simulink model "motor_unit"  (Simulink 7.8)
settings: Solver=ode14x  StartTime=0.0  StopTime=1  FixedStep=0.001  RelTol=1e-3
InitFcn:
  | [A tau T] = emg_filter()
  | [A_twitch T_twitch tau_twitch P e] = twitch_filter()
  |  [mag1 mag2 A_rise A_fall T] = get_active_function_coeff()
  | set_trfcn()
StopFcn:
  | incrementVars('motor_unit')
values from neighbouring files (symbols this model uses):
  A = exp(-T/tau)    [emg_filter.m]    (also in twitch_filter.m = [1 -2*A_twitch A_twitch^2] * P * e * A_twitch / tau_twitch)
  A_rise = exp(-T/t_rise)    [get_active_function_coeff.m]    (also in set_mu.m; set_mu_spasticity.m; set_trfcn.m)
  mag1 = 318144    [get_active_function_coeff.m]    (also in set_mu.m; set_mu_spasticity.m; set_trfcn.m)
  mag2 = 45845    [get_active_function_coeff.m]    (also in set_mu.m; set_mu_spasticity.m; set_trfcn.m)
  T = 1/1024    (= 0.0009765625)    [emg_filter.m]    (also in get_active_function_coeff.m = 0.001; set_mu.m = 0.001; set_mu_spasticity.m = 0.001; set_trfcn.m = 0.001)
  tau = 0.008    [emg_filter.m]
undefined symbols (not defined in the file or in its folder): dfilt, fdesignblkfcn, gcbh
libraries: cstblocks x25, simulink x11, dsparch4 x3
settings Model: Creator=minos_niu  LastModifiedBy=PXI_BBDL
settings DebuggingCC: FcnCallInpInsideContextMsg=Use local settings

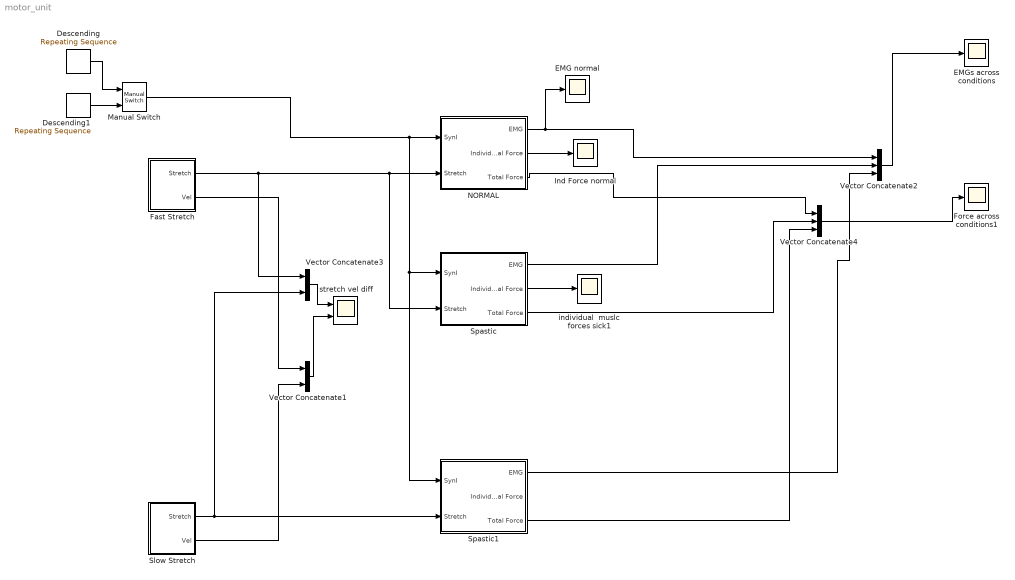
== system motor_unit ==
  Descending : simulink/Sources/Repeating Sequence  rep_seq_t=[0 0.5 1]  rep_seq_y=[0 200 200]*1
  Descending1 : simulink/Sources/Repeating Sequence  rep_seq_t=[0 0.5 1]  rep_seq_y=[0 200 200]*0
  EMG normal : Scope
      settings: TickLabels=on  TimeRange=1  YMin=-1000  YMax=5000  SaveName=ScopeData24
  EMGs across conditions : Scope
      settings: TickLabels=on  TimeRange=1  YMin=-1000  YMax=5000  SaveName=ScopeData6
  Fast Stretch : Subsystem
  Force across conditions1 : Scope
      settings: TickLabels=on  TimeRange=1  YMin=-1000  YMax=5000  SaveName=ScopeData5
  Ind Force normal : Scope
      settings: TickLabels=on  TimeRange=1  YMin=0  YMax=9e+09  SaveName=ScopeData21
  Manual Switch : simulink/Signal Routing/Manual Switch  sw=0  action=0  varsize=off
  NORMAL : Subsystem
  Slow Stretch : Subsystem
  Spastic : Subsystem
  Spastic1 : Subsystem
  Vector Concatenate1 : Concatenate  Mode=Vector
  Vector Concatenate2 : Concatenate  NumInputs=3  Mode=Vector
  Vector Concatenate3 : Concatenate  Mode=Vector
  Vector Concatenate4 : Concatenate  NumInputs=3  Mode=Vector
  individual  muslc forces sick1 : Scope
      settings: TickLabels=on  TimeRange=1  YMin=0  YMax=1.4e+10  SaveName=ScopeData8
  stretch vel diff : Scope  NumInputPorts=2
      settings: TickLabels=on  TimeRange=1  YMin=-5~-5  YMax=5~5  SaveName=ScopeData41
  wires:
  Spastic/1(EMG) -> Vector Concatenate2/2
  NORMAL/1(EMG) -> Vector Concatenate2/1, EMG normal/1
  NORMAL/3(Total Force) -> Vector Concatenate4/1
  Spastic/2(Individual Force) -> individual  muslc forces sick1/1
  Spastic/3(Total Force) -> Vector Concatenate4/2
  Vector Concatenate4/1 -> Force across conditions1/1
  Vector Concatenate2/1 -> EMGs across conditions/1
  Vector Concatenate1/1 -> stretch vel diff/2
  Vector Concatenate3/1 -> stretch vel diff/1
  Fast Stretch/1(Stretch) -> NORMAL/2(Stretch), Spastic/2(Stretch), Vector Concatenate3/1
  Slow Stretch/1(Stretch) -> Spastic1/2(Stretch), Vector Concatenate3/2
  Spastic1/1(EMG) -> Vector Concatenate2/3
  Fast Stretch/2(Vel) -> Vector Concatenate1/1
  Slow Stretch/2(Vel) -> Vector Concatenate1/2
  NORMAL/2(Individual Force) -> Ind Force normal/1
  Spastic1/3(Total Force) -> Vector Concatenate4/3
  Manual Switch/1 -> NORMAL/1(SynI), Spastic/1(SynI), Spastic1/1(SynI)
  Descending/1 -> Manual Switch/1
  Descending1/1 -> Manual Switch/2

== system motor_unit/Fast Stretch ==
  Discrete Derivative : simulink/Discrete/Discrete Derivative  gainval=1.0  ICPrevScaledInput=0.0  InputProcessing=Inherited  OutMin=[]  OutMax=[]  OutDataType=fixdt(1, 16)  OutScaling=2^-10  DoSatur=off
  Manual Switch : simulink/Signal Routing/Manual Switch  sw=0  action=0  varsize=off
  muscle stretch : simulink/Sources/Repeating Sequence  rep_seq_t=[0 0.25 0.8 1.5]  rep_seq_y=[1 1.00 1.0 1.0]
  muscle stretch1 : simulink/Sources/Repeating Sequence  rep_seq_t=[0 0.25 0.8 1.5]  rep_seq_y=[1 1.00 1.5 1.5]
  Stretch : Outport
  Vel : Outport  Port=2
  wires:
  Discrete Derivative/1 -> Vel/1
  Manual Switch/1 -> Discrete Derivative/1, Stretch/1
  muscle stretch/1 -> Manual Switch/1
  muscle stretch1/1 -> Manual Switch/2

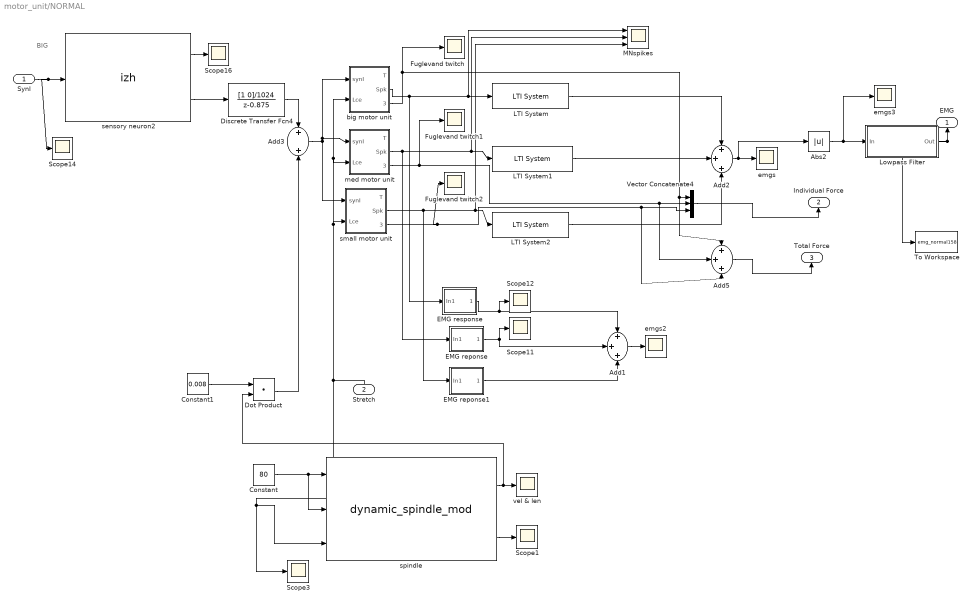
== system motor_unit/NORMAL ==
  note: BIG
  SynI : Inport
  Stretch : Inport  Port=2
  Abs2 : Abs
  Add1 : Sum  Inputs=+++
  Add2 : Sum  Inputs=+++
  Add3 : Sum
  Add5 : Sum  Inputs=+++
  Constant : Constant  Value=80
  Constant1 : Constant  Value=0.008
  Discrete Transfer Fcn4 : DiscreteTransferFcn  Numerator=[1 0]/1024  Denominator=[1 -0.875]  SampleTime=0.001
  Dot Product : DotProduct  InputSameDT=on  OutDataTypeStr=Inherit: Inherit via internal rule
  EMG reponse : Subsystem
  EMG reponse1 : Subsystem
  EMG response : Subsystem
  Fuglevand twitch : Scope
      settings: YMin=0  YMax=225
  Fuglevand twitch1 : Scope
      settings: YMin=0  YMax=225  SaveName=ScopeData27
  Fuglevand twitch2 : Scope
      settings: YMin=0  YMax=225  SaveName=ScopeData28
  LTI System : cstblocks/LTI System  sys=zpk([0], [A A], 2*T*A, T) - zpk([0 -A], [A A A], T^2*A/tau, T)  IC=[]
  LTI System1 : cstblocks/LTI System  sys=zpk([0], [A A], 2*T*A, T) - zpk([0 -A], [A A A], T^2*A/tau, T)  IC=[]
  LTI System2 : cstblocks/LTI System  sys=zpk([0], [A A], 2*T*A, T) - zpk([0 -A], [A A A], T^2*A/tau, T)  IC=[]
  Lowpass Filter : Subsystem  DialogController=fdesignblkfcn  DialogControllerArgs=DataTag1  InitFcn=fdesignblkfcn(gcbh, {'InitFcn'});
      settings: CopyFcn=fdesignblkfcn(gcbh, {'CopyFcn'});
      mask Type: Lowpass Filter
      mask Description: Design a lowpass filter
      mask Help: helpview(mapfilelocation('dsp'), 'dsplowpassfilter');
      mask Display: disp('Lowpass')
  MNspikes : Scope  NumInputPorts=3
      settings: YMin=0~-5~-5  YMax=225~5~5  SaveName=ScopeData2
  Scope{1,3,11..12,14,16} (6 alike) : Scope
      Scope1 settings: TimeRange=1  SaveName=ScopeData17
      Scope11 settings: SaveName=ScopeData9
      Scope12 settings: SaveName=ScopeData13
      Scope14 settings: YMin=0  YMax=225  SaveName=ScopeData14
      Scope16 settings: SaveName=ScopeData16
      Scope3 settings: SaveName=ScopeData18
  To Workspace : ToWorkspace  VariableName=emg_normal158  SampleTime=-1  SaveFormat=Structure With Time
  Vector Concatenate4 : Concatenate  NumInputs=3  Mode=Vector
  big motor unit : Subsystem
  emgs : Scope
      settings: YMin=0  YMax=225
  emgs2 : Scope
      settings: TimeRange=1  YMin=-0.03  YMax=0.03  SaveName=ScopeData15
  emgs3 : Scope
      settings: YMin=0  YMax=225  SaveName=ScopeData3
  med motor unit : Subsystem
  sensory neuron2 : S-Function  FunctionName=izh  Parameters=[0.02 0.2 -65.0 6.0 30.0 3.0] [-70.0 -14.0]  EnableBusSupport=off
      mask Display:
      | port_label('input', 1, 'syn curr');
      | port_label('output', 1, 'action potential');
      | port_label('output', 2, 'spike');
      | disp('Izhi Neuron \n(S-Function)')
  small motor unit : Subsystem
  spindle : S-Function  FunctionName=dynamic_spindle_mod  Parameters=[10.4649 10.4649 10.4649] [0.1127 0.1623 0.1623] [0.0605 0.0822 0.0822] [0.2356 -0.046 -0.069] [0 0 0] [0.0289 0.0636 0.0954] [1 0.7 0.7] [1 0.92 0.92] [20000 10000 10000] [20000 7250 7250] [0.3 0.3 0.3] [0.46 0.46 0.46] [0.04 0.04 0.04] [0.76 0.76 0.76] [1 0.04 0.04] [0.192 0.185 0.0001] [0.0002 0.0002 0.0002] [1 0.5 1] [1]  EnableBusSupport=off
      mask Display:
      | port_label('input', 1, 'gamma dynamic');
      | port_label('input', 2, 'gamma static');
      | port_label('input', 3, 'Lce(L0)');
      | port_label('output',1,'Ia');
      | port_label('output',2,'II');
      | disp('Muscle Spindle \n(S-Function)')
  vel & len : Scope
      settings: SaveName=ScopeData12
  EMG : Outport
  Individual Force : Outport  Port=2
  Total Force : Outport  Port=3
  wires:
  Abs2/1 -> Lowpass Filter/1(In), emgs3/1
  Lowpass Filter/1(Out) -> To Workspace/1, EMG/1
  Add3/1 -> big motor unit/1(synI), med motor unit/1(synI), small motor unit/1(synI)
  Discrete Transfer Fcn4/1 -> Add3/1
  Dot Product/1 -> Add3/2
  Constant1/1 -> Dot Product/1
  Stretch/1 -> Scope3/1, spindle/3, big motor unit/2(Lce), med motor unit/2(Lce), small motor unit/2(Lce)
  spindle/2 -> Scope1/1
  spindle/1 -> vel & len/1, Dot Product/2
  Constant/1 -> spindle/1, spindle/2
  EMG reponse1/1(Out1) -> Add1/3
  Add1/1 -> emgs2/1
  big motor unit/2(Spk) -> EMG response/1(In1), LTI System/1, MNspikes/1
  LTI System2/1 -> Add2/3
  LTI System1/1 -> Add2/2
  LTI System/1 -> Add2/1
  Add2/1 -> emgs/1, Abs2/1
  sensory neuron2/2 -> Discrete Transfer Fcn4/1
  Add5/1 -> Total Force/1
  sensory neuron2/1 -> Scope16/1
  SynI/1 -> Scope14/1, sensory neuron2/1
  EMG response/1(Out1) -> Scope12/1, Add1/1
  EMG reponse/1(Out1) -> Scope11/1, Add1/2
  Vector Concatenate4/1 -> Individual Force/1
  big motor unit/3(Fubglevant  twitch normal) -> Fuglevand twitch/1, Vector Concatenate4/1, Add5/1
  med motor unit/2(Spk) -> EMG reponse/1(In1), LTI System1/1, MNspikes/2
  small motor unit/2(Spk) -> EMG reponse1/1(In1), LTI System2/1, MNspikes/3
  med motor unit/3(Fubglevant  twitch normal) -> Fuglevand twitch1/1, Vector Concatenate4/2, Add5/2
  small motor unit/3(Fubglevant  twitch normal) -> Fuglevand twitch2/1, Vector Concatenate4/3, Add5/3

== system motor_unit/Slow Stretch ==
  Discrete Derivative : simulink/Discrete/Discrete Derivative  gainval=1.0  ICPrevScaledInput=0.0  InputProcessing=Inherited  OutMin=[]  OutMax=[]  OutDataType=fixdt(1, 16)  OutScaling=2^-10  DoSatur=off
  Manual Switch : simulink/Signal Routing/Manual Switch  sw=0  action=0  varsize=off
  muscle stretch : simulink/Sources/Repeating Sequence  rep_seq_t=[0 0.25 0.8 1.5]  rep_seq_y=[1 1.00 1.0 1.0]
  muscle stretch1 : simulink/Sources/Repeating Sequence  rep_seq_t=[0 0.25 0.65 1.5]  rep_seq_y=[1 1.00 1.5 1.5]
  Stretch : Outport
  Vel : Outport  Port=2
  wires:
  muscle stretch1/1 -> Manual Switch/2
  muscle stretch/1 -> Manual Switch/1
  Manual Switch/1 -> Stretch/1, Discrete Derivative/1
  Discrete Derivative/1 -> Vel/1

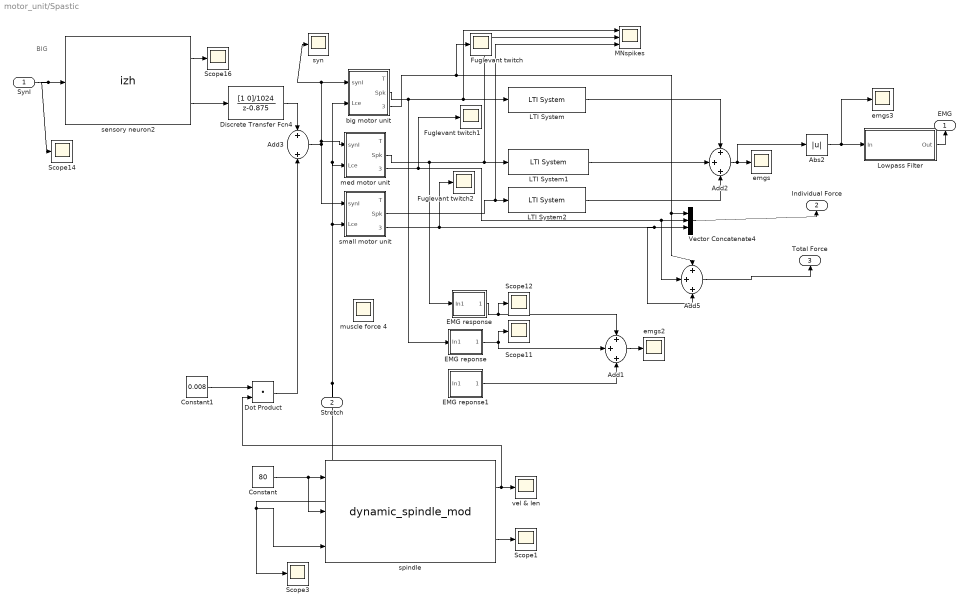
== system motor_unit/Spastic ==
  note: BIG
  SynI : Inport
  Stretch : Inport  Port=2
  " Fuglevant twitch" : Scope
      settings: YMin=0  YMax=225  SaveName=ScopeData26
  " Fuglevant twitch1" : Scope
      settings: YMin=0  YMax=225  SaveName=ScopeData4
  " Fuglevant twitch2" : Scope
      settings: YMin=0  YMax=225  SaveName=ScopeData11
  Abs2 : Abs
  Add1 : Sum  Inputs=+++
  Add2 : Sum  Inputs=+++
  Add3 : Sum
  Add5 : Sum  Inputs=+++
  Constant : Constant  Value=80
  Constant1 : Constant  Value=0.008
  Discrete Transfer Fcn4 : DiscreteTransferFcn  Numerator=[1 0]/1024  Denominator=[1 -0.875]  SampleTime=0.001
  Dot Product : DotProduct  InputSameDT=on  OutDataTypeStr=Inherit: Inherit via internal rule
  EMG reponse : Subsystem
  EMG reponse1 : Subsystem
  EMG response : Subsystem
  LTI System : cstblocks/LTI System  sys=zpk([0], [A A], 2*T*A, T) - zpk([0 -A], [A A A], T^2*A/tau, T)  IC=[]
  LTI System1 : cstblocks/LTI System  sys=zpk([0], [A A], 2*T*A, T) - zpk([0 -A], [A A A], T^2*A/tau, T)  IC=[]
  LTI System2 : cstblocks/LTI System  sys=zpk([0], [A A], 2*T*A, T) - zpk([0 -A], [A A A], T^2*A/tau, T)  IC=[]
  Lowpass Filter : Subsystem  DialogController=fdesignblkfcn  DialogControllerArgs=DataTag4  InitFcn=fdesignblkfcn(gcbh, {'InitFcn'});
      settings: CopyFcn=fdesignblkfcn(gcbh, {'CopyFcn'});
      mask Type: Lowpass Filter
      mask Description: Design a lowpass filter
      mask Help: helpview(mapfilelocation('dsp'), 'dsplowpassfilter');
      mask Display: disp('Lowpass')
  MNspikes : Scope  NumInputPorts=3
      settings: YMin=0~-5~-5  YMax=225~5~5  SaveName=ScopeData20
  Scope{1,3,11..12,14,16} (6 alike) : Scope
      Scope1 settings: TimeRange=1  SaveName=ScopeData17
      Scope11 settings: SaveName=ScopeData9
      Scope12 settings: SaveName=ScopeData13
      Scope14 settings: YMin=0  YMax=225  SaveName=ScopeData14
      Scope16 settings: SaveName=ScopeData16
      Scope3 settings: SaveName=ScopeData18
  Vector Concatenate4 : Concatenate  NumInputs=3  Mode=Vector
  big motor unit : Subsystem
  emgs : Scope
      settings: YMin=0  YMax=225
  emgs2 : Scope
      settings: TimeRange=1  YMin=-0.03  YMax=0.03  SaveName=ScopeData15
  emgs3 : Scope
      settings: YMin=0  YMax=225  SaveName=ScopeData3
  med motor unit : Subsystem
  muscle force 4 : Scope
      settings: YMin=0  YMax=225  SaveName=ScopeData7
  sensory neuron2 : S-Function  FunctionName=izh  Parameters=[0.02 0.2 -65.0 6.0 30.0 3.0] [-70.0 -14.0]  EnableBusSupport=off
      mask Display:
      | port_label('input', 1, 'syn curr');
      | port_label('output', 1, 'action potential');
      | port_label('output', 2, 'spike');
      | disp('Izhi Neuron \n(S-Function)')
  small motor unit : Subsystem
  spindle : S-Function  FunctionName=dynamic_spindle_mod  Parameters=[10.4649 10.4649 10.4649] [0.1127 0.1623 0.1623] [0.0605 0.0822 0.0822] [0.2356 -0.046 -0.069] [0 0 0] [0.0289 0.0636 0.0954] [1 0.7 0.7] [1 0.92 0.92] [20000 10000 10000] [20000 7250 7250] [0.3 0.3 0.3] [0.46 0.46 0.46] [0.04 0.04 0.04] [0.76 0.76 0.76] [1 0.04 0.04] [0.192 0.185 0.0001] [0.0002 0.0002 0.0002] [1 0.5 1] [1]  EnableBusSupport=off
      mask Display:
      | port_label('input', 1, 'gamma dynamic');
      | port_label('input', 2, 'gamma static');
      | port_label('input', 3, 'Lce(L0)');
      | port_label('output',1,'Ia');
      | port_label('output',2,'II');
      | disp('Muscle Spindle \n(S-Function)')
  syn : Scope
      settings: YMin=0  YMax=225  SaveName=ScopeData25
  vel & len : Scope
      settings: SaveName=ScopeData12
  EMG : Outport
  Individual Force : Outport  Port=2
  Total Force : Outport  Port=3
  wires:
  Vector Concatenate4/1 -> Individual Force/1
  EMG reponse/1(Out1) -> Add1/2, Scope11/1
  EMG response/1(Out1) -> Add1/1, Scope12/1
  SynI/1 -> sensory neuron2/1, Scope14/1
  sensory neuron2/1 -> Scope16/1
  Add5/1 -> Total Force/1
  sensory neuron2/2 -> Discrete Transfer Fcn4/1
  Add2/1 -> Abs2/1, emgs/1
  LTI System/1 -> Add2/1
  LTI System1/1 -> Add2/2
  LTI System2/1 -> Add2/3
  big motor unit/2(Spk) -> EMG reponse/1(In1), LTI System/1, MNspikes/1
  med motor unit/2(Spk) -> EMG response/1(In1), LTI System1/1, MNspikes/2
  Add1/1 -> emgs2/1
  EMG reponse1/1(Out1) -> Add1/3
  Constant/1 -> spindle/2, spindle/1
  spindle/1 -> Dot Product/2, vel & len/1
  spindle/2 -> Scope1/1
  Stretch/1 -> spindle/3, Scope3/1, big motor unit/2(Lce), med motor unit/2(Lce), small motor unit/2(Lce)
  Constant1/1 -> Dot Product/1
  Dot Product/1 -> Add3/2
  Discrete Transfer Fcn4/1 -> Add3/1
  Add3/1 -> big motor unit/1(synI), syn/1, med motor unit/1(synI), small motor unit/1(synI)
  Lowpass Filter/1(Out) -> EMG/1
  Abs2/1 -> emgs3/1, Lowpass Filter/1(In)
  med motor unit/3(Fubglevant  twitch) -> Vector Concatenate4/2, Add5/2, " Fuglevant twitch1"/1
  big motor unit/3(Fubglevant  twitch) -> " Fuglevant twitch"/1, Vector Concatenate4/1, Add5/1
  small motor unit/3(Fubglevant  twitch) -> Vector Concatenate4/3, Add5/3, " Fuglevant twitch2"/1
  small motor unit/2(Spk) -> LTI System2/1, MNspikes/3

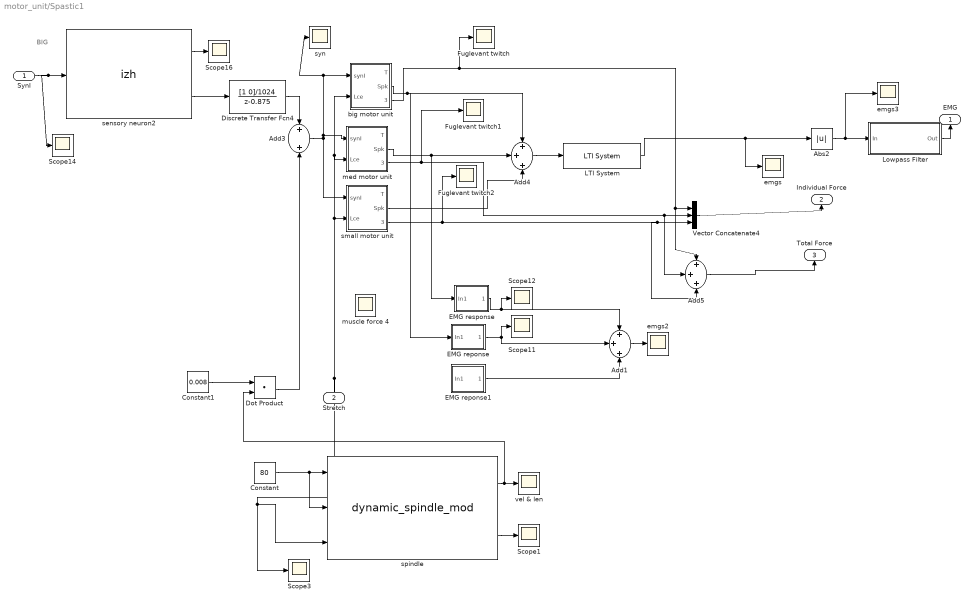
== system motor_unit/Spastic1 ==
  note: BIG
  SynI : Inport
  Stretch : Inport  Port=2
  " Fuglevant twitch" : Scope
      settings: YMin=0  YMax=225  SaveName=ScopeData26
  " Fuglevant twitch1" : Scope
      settings: YMin=0  YMax=225  SaveName=ScopeData4
  " Fuglevant twitch2" : Scope
      settings: YMin=0  YMax=225  SaveName=ScopeData11
  Abs2 : Abs
  Add1 : Sum  Inputs=+++
  Add3 : Sum
  Add4 : Sum  Inputs=+++
  Add5 : Sum  Inputs=+++
  Constant : Constant  Value=80
  Constant1 : Constant  Value=0.008
  Discrete Transfer Fcn4 : DiscreteTransferFcn  Numerator=[1 0]/1024  Denominator=[1 -0.875]  SampleTime=0.001
  Dot Product : DotProduct  InputSameDT=on  OutDataTypeStr=Inherit: Inherit via internal rule
  EMG reponse : Subsystem
  EMG reponse1 : Subsystem
  EMG response : Subsystem
  LTI System : cstblocks/LTI System  sys=zpk([0], [A A], 2*T*A, T) - zpk([0 -A], [A A A], T^2*A/tau, T)  IC=[]
  Lowpass Filter : Subsystem  DialogController=fdesignblkfcn  DialogControllerArgs=DataTag7  InitFcn=fdesignblkfcn(gcbh, {'InitFcn'});
      settings: CopyFcn=fdesignblkfcn(gcbh, {'CopyFcn'});
      mask Type: Lowpass Filter
      mask Description: Design a lowpass filter
      mask Help: helpview(mapfilelocation('dsp'), 'dsplowpassfilter');
      mask Display: disp('Lowpass')
  Scope{1,3,11..12,14,16} (6 alike) : Scope
      Scope1 settings: TimeRange=1  SaveName=ScopeData17
      Scope11 settings: SaveName=ScopeData9
      Scope12 settings: SaveName=ScopeData13
      Scope14 settings: YMin=0  YMax=225  SaveName=ScopeData14
      Scope16 settings: SaveName=ScopeData16
      Scope3 settings: SaveName=ScopeData18
  Vector Concatenate4 : Concatenate  NumInputs=3  Mode=Vector
  big motor unit : Subsystem
  emgs : Scope
      settings: YMin=0  YMax=225
  emgs2 : Scope
      settings: TimeRange=1  YMin=-0.03  YMax=0.03  SaveName=ScopeData15
  emgs3 : Scope
      settings: YMin=0  YMax=225  SaveName=ScopeData3
  med motor unit : Subsystem
  muscle force 4 : Scope
      settings: YMin=0  YMax=225  SaveName=ScopeData7
  sensory neuron2 : S-Function  FunctionName=izh  Parameters=[0.02 0.2 -65.0 6.0 30.0 3.0] [-70.0 -14.0]  EnableBusSupport=off
      mask Display:
      | port_label('input', 1, 'syn curr');
      | port_label('output', 1, 'action potential');
      | port_label('output', 2, 'spike');
      | disp('Izhi Neuron \n(S-Function)')
  small motor unit : Subsystem
  spindle : S-Function  FunctionName=dynamic_spindle_mod  Parameters=[10.4649 10.4649 10.4649] [0.1127 0.1623 0.1623] [0.0605 0.0822 0.0822] [0.2356 -0.046 -0.069] [0 0 0] [0.0289 0.0636 0.0954] [1 0.7 0.7] [1 0.92 0.92] [20000 10000 10000] [20000 7250 7250] [0.3 0.3 0.3] [0.46 0.46 0.46] [0.04 0.04 0.04] [0.76 0.76 0.76] [1 0.04 0.04] [0.192 0.185 0.0001] [0.0002 0.0002 0.0002] [1 0.5 1] [1]  EnableBusSupport=off
      mask Display:
      | port_label('input', 1, 'gamma dynamic');
      | port_label('input', 2, 'gamma static');
      | port_label('input', 3, 'Lce(L0)');
      | port_label('output',1,'Ia');
      | port_label('output',2,'II');
      | disp('Muscle Spindle \n(S-Function)')
  syn : Scope
      settings: YMin=0  YMax=225  SaveName=ScopeData25
  vel & len : Scope
      settings: SaveName=ScopeData12
  EMG : Outport
  Individual Force : Outport  Port=2
  Total Force : Outport  Port=3
  wires:
  small motor unit/2(Spk) -> Add4/3
  small motor unit/3(Fubglevant  twitch) -> " Fuglevant twitch2"/1, Add5/3, Vector Concatenate4/3
  big motor unit/3(Fubglevant  twitch) -> Add5/1, Vector Concatenate4/1, " Fuglevant twitch"/1
  med motor unit/3(Fubglevant  twitch) -> " Fuglevant twitch1"/1, Add5/2, Vector Concatenate4/2
  Abs2/1 -> Lowpass Filter/1(In), emgs3/1
  Lowpass Filter/1(Out) -> EMG/1
  Add3/1 -> small motor unit/1(synI), med motor unit/1(synI), syn/1, big motor unit/1(synI)
  Discrete Transfer Fcn4/1 -> Add3/1
  Dot Product/1 -> Add3/2
  Constant1/1 -> Dot Product/1
  Stretch/1 -> small motor unit/2(Lce), med motor unit/2(Lce), big motor unit/2(Lce), Scope3/1, spindle/3
  spindle/2 -> Scope1/1
  spindle/1 -> vel & len/1, Dot Product/2
  Constant/1 -> spindle/1, spindle/2
  EMG reponse1/1(Out1) -> Add1/3
  Add1/1 -> emgs2/1
  med motor unit/2(Spk) -> EMG response/1(In1), Add4/2
  big motor unit/2(Spk) -> EMG reponse/1(In1), Add4/1
  LTI System/1 -> emgs/1, Abs2/1
  sensory neuron2/2 -> Discrete Transfer Fcn4/1
  Add5/1 -> Total Force/1
  sensory neuron2/1 -> Scope16/1
  SynI/1 -> Scope14/1, sensory neuron2/1
  EMG response/1(Out1) -> Scope12/1, Add1/1
  EMG reponse/1(Out1) -> Scope11/1, Add1/2
  Vector Concatenate4/1 -> Individual Force/1
  Add4/1 -> LTI System/1

== system motor_unit/NORMAL/EMG reponse ==
  In1 : Inport
  Add1 : Sum
  Zero-Pole : ZeroPole  Zeros=[]  Poles=[-33 -33]  Gain=[2]
  Zero-Pole1 : ZeroPole  Zeros=[]  Poles=[-33 -33 -33]  Gain=[-2 * 33]
  Out1 : Outport
  wires:
  Zero-Pole/1 -> Add1/1
  Zero-Pole1/1 -> Add1/2
  Add1/1 -> Out1/1
  In1/1 -> Zero-Pole/1, Zero-Pole1/1

== system motor_unit/NORMAL/EMG reponse1 ==
  In1 : Inport
  Add1 : Sum
  Zero-Pole : ZeroPole  Zeros=[]  Poles=[-33 -33]  Gain=[2]
  Zero-Pole1 : ZeroPole  Zeros=[]  Poles=[-33 -33 -33]  Gain=[-2 * 33]
  Out1 : Outport
  wires:
  Zero-Pole/1 -> Add1/1
  Zero-Pole1/1 -> Add1/2
  Add1/1 -> Out1/1
  In1/1 -> Zero-Pole/1, Zero-Pole1/1

== system motor_unit/NORMAL/EMG response ==
  In1 : Inport
  Add2 : Sum
  Zero-Pole2 : ZeroPole  Zeros=[]  Poles=[-33 -33]  Gain=[2]
  Zero-Pole3 : ZeroPole  Zeros=[]  Poles=[-33 -33 -33]  Gain=[-2 * 33]
  Out1 : Outport
  wires:
  Zero-Pole3/1 -> Add2/2
  Zero-Pole2/1 -> Add2/1
  In1/1 -> Zero-Pole2/1, Zero-Pole3/1
  Add2/1 -> Out1/1

== system motor_unit/NORMAL/Lowpass Filter ==
  In : Inport
  Generated Filter Block : dsparch4/Digital Filter  Tag=BlockMethodSubSystem  TypePopup=FIR (all zeros)  IIRFiltStruct=Direct form II transposed  AllPoleFiltStruct=Direct form  FIRFiltStruct=Direct form  CoeffSource=Specify via dialog  NumCoeffs=[0.000821343113298559 0.000860441837741389 0.00116507777294478 0.00139896051971534 0.00148073798259756 0.00133051719232521 0.000881379928818246 9.39666659446496e-05 -0.00102427649336678 -0.00241508381296073 -0.00396005761838719 -0.00548791113381279 -0.00678957165103652 -0.0076430176358472 -0.00784363593055865 -0.00724034355165257 -0.005767373855361 -0.00347179427273649 -0.000526738025008324 0.00277189505493066 0.00602772399348037 0.00878384411363102 0.0105793849551558 0.0110144101671425 0.00981730876000813 0.00690368741433792 0.00241805574190362 -0.00324979313849789 -0.00947842883556182 -0.0154612118882062 -0.0202815328070714 -0.0230109852998383 -0.0228194406688834 -0.0190843479651619 -0.0114852033107793 -7.04588646032898e-05 0.0147140504913441 0.032040450344853 0.0507590050669597 0.0694980891161205 0.0867940010093986 0.101236365407667 0.111612741087645 0.117035389882844 0.117035389882844 0.111612741087645 0.101236365407667 0.0867940010093986 0.0694980891161205 0.0507590050669597 0.032040450344853 0.0147140504913441 -7.04588646032898e-05 -0.0114852033107793 -0.0190843479651619 -0.0228194406688834 -0.0230109852998383 -0.0202815328070714 -0.0154612118882062 -0.00947842883556182 -0.00324979313849789 0.00241805574190362 0.00690368741433792 0.00981730876000813 0.0110144101671425 0.0105793849551558 0.00878384411363102 0.00602772399348037 0.00277189505493066 -0.000526738025008324 -0.00347179427273649 -0.005767373855361 -0.00724034355165257 -0.00784363593055865 -0.0076430176358472 -0.00678957165103652 -0.00548791113381279 -0.00396005761838719 -0.00241508381296073 -0.00102427649336678 9.39666659446496e-05 0.000881379928818246 0.00133051719232521 0.00148073798259756 0.00139896051971534 0.00116507777294478 0.000860441837741389 0.000821343113298559]  DenCoeffs=[1 0.1]  BiQuadCoeffs=[1 0.3 0.4 1 0.1 0.2]  LatticeCoeffs=[0.2 0.4]  denIgnore=on  FiltPerSampPopup=One filter per frame  IC=0  ICnum=0  ICden=0  roundingMode=Floor  overflowMode=off  ScaleValues=1  scaleValueFracLength=14  stageInFracLength=15  stageOutFracLength=15  FilterSource=Specify via dialog  dfiltObjectName=dfilt.dffir([1 2 1])  InputProcessing=Columns as channels (frame based)
  Out : Outport
  wires:
  In/1 -> Generated Filter Block/1
  Generated Filter Block/1 -> Out/1

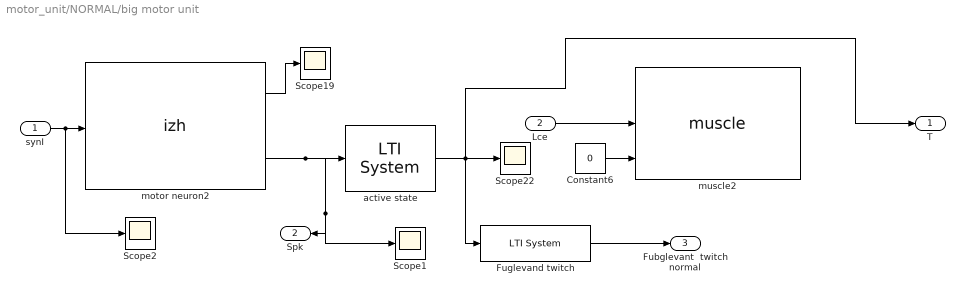
== system motor_unit/NORMAL/big motor unit ==
  synI : Inport
  Lce : Inport  Port=2
  Constant6 : Constant  Value=0
  Fuglevand twitch : cstblocks/LTI System  sys=zpk([0], [0.93941 0.93941], 1*2.7183*0.001*0.93941/0.016, 0.001)  IC=[]
  Scope{1..2,19,22} (4 alike) : Scope
      Scope1 settings: TimeRange=0.4  YMin=-1000  YMax=5000  SaveName=ScopeData10
      Scope19 settings: SaveName=ScopeData19
      Scope2 settings: SaveName=ScopeData29
      Scope22 settings: TimeRange=0.4  YMin=-1000  YMax=5000  SaveName=ScopeData22
  active state : cstblocks/LTI System  sys="0*zpk([0], 0.97531, 318144, T) + zpk([0], exp(-T/0.04),  mag2*8, T)"  IC=[]
  motor neuron2 : S-Function  FunctionName=izh  Parameters=[0.02 0.2 -65.0 6.0 30.0 0.45] [-70.0 -14.0]  EnableBusSupport=off
      mask Display:
      | port_label('input', 1, 'syn curr');
      | port_label('output', 1, 'action potential');
      | port_label('output', 2, 'spike');
      | disp('Izhi Neuron \n(S-Function)')
  muscle2 : S-Function  FunctionName=muscle  Parameters=[136.0 75.0 50.0] [0]  EnableBusSupport=off
      mask Display:
      | port_label('input', 1, 'Active state');
      | port_label('input', 2, 'length');
      | port_label('input', 3, 'vel');
      | port_label('output', 1, 'tension');
      | disp('muscle model \n(S-Function)');
  T : Outport
  Spk : Outport  Port=2
  Fubglevant  twitch normal : Outport  Port=3
  wires:
  Constant6/1 -> muscle2/3
  motor neuron2/1 -> Scope19/1
  active state/1 -> Scope22/1, T/1, Fuglevand twitch/1
  motor neuron2/2 -> active state/1, Spk/1, Scope1/1
  synI/1 -> motor neuron2/1, Scope2/1
  Lce/1 -> muscle2/2
  Fuglevand twitch/1 -> Fubglevant  twitch normal/1

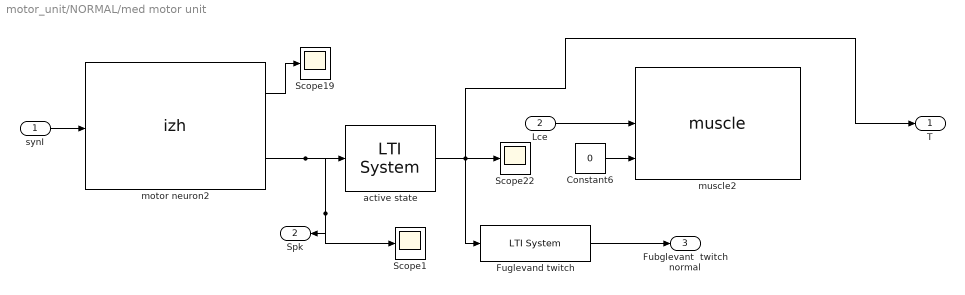
== system motor_unit/NORMAL/med motor unit ==
  synI : Inport
  Lce : Inport  Port=2
  Constant6 : Constant  Value=0
  Fuglevand twitch : cstblocks/LTI System  sys=zpk([0], [0.93941 0.93941], 1*2.7183*0.001*0.93941/0.016, 0.001)  IC=[]
  Scope1 : Scope
      settings: TimeRange=0.4  YMin=-1000  YMax=5000  SaveName=ScopeData10
  Scope19 : Scope
      settings: SaveName=ScopeData19
  Scope22 : Scope
      settings: TimeRange=0.4  YMin=-1000  YMax=5000  SaveName=ScopeData22
  active state : cstblocks/LTI System  sys="0*zpk([0], A_rise, mag1, T) + zpk([0], exp(-T/0.06),  mag2*3.5, T)"  IC=[]
  motor neuron2 : S-Function  FunctionName=izh  Parameters=[0.02 0.2 -65.0 6.0 30.0 0.50] [-70.0 -14.0]  EnableBusSupport=off
      mask Display:
      | port_label('input', 1, 'syn curr');
      | port_label('output', 1, 'action potential');
      | port_label('output', 2, 'spike');
      | disp('Izhi Neuron \n(S-Function)')
  muscle2 : S-Function  FunctionName=muscle  Parameters=[136.0 75.0 50.0] [0]  EnableBusSupport=off
      mask Display:
      | port_label('input', 1, 'Active state');
      | port_label('input', 2, 'length');
      | port_label('input', 3, 'vel');
      | port_label('output', 1, 'tension');
      | disp('muscle model \n(S-Function)');
  T : Outport
  Spk : Outport  Port=2
  Fubglevant  twitch normal : Outport  Port=3
  wires:
  Fuglevand twitch/1 -> Fubglevant  twitch normal/1
  Lce/1 -> muscle2/2
  synI/1 -> motor neuron2/1
  motor neuron2/2 -> Scope1/1, Spk/1, active state/1
  active state/1 -> Fuglevand twitch/1, T/1, Scope22/1
  motor neuron2/1 -> Scope19/1
  Constant6/1 -> muscle2/3

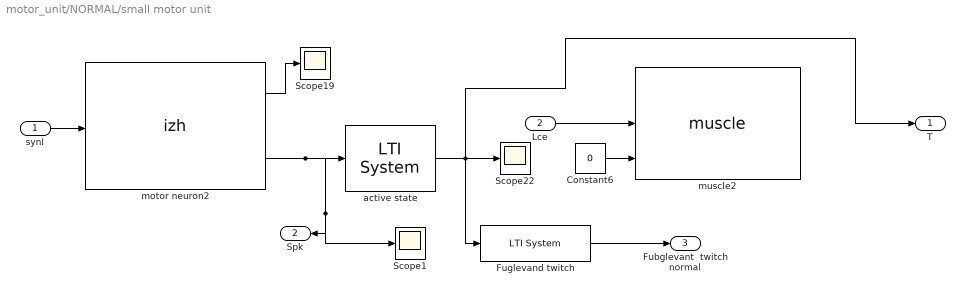
== system motor_unit/NORMAL/small motor unit ==
  synI : Inport
  Lce : Inport  Port=2
  Constant6 : Constant  Value=0
  Fuglevand twitch : cstblocks/LTI System  sys=zpk([0], [0.93941 0.93941], 1*2.7183*0.001*0.93941/0.016, 0.001)  IC=[]
  Scope1 : Scope
      settings: TimeRange=0.4  YMin=-1000  YMax=5000  SaveName=ScopeData10
  Scope19 : Scope
      settings: SaveName=ScopeData19
  Scope22 : Scope
      settings: TimeRange=0.4  YMin=-1000  YMax=5000  SaveName=ScopeData22
  active state : cstblocks/LTI System  sys=0*zpk([0], A_rise, mag1, T) + zpk([0], exp(-T/0.09), mag2*1, T)  IC=[]
  motor neuron2 : S-Function  FunctionName=izh  Parameters=[0.02 0.2 -65.0 6.0 30.0 0.55] [-70.0 -14.0]  EnableBusSupport=off
      mask Display:
      | port_label('input', 1, 'syn curr');
      | port_label('output', 1, 'action potential');
      | port_label('output', 2, 'spike');
      | disp('Izhi Neuron \n(S-Function)')
  muscle2 : S-Function  FunctionName=muscle  Parameters=[136.0 75.0 50.0] [0]  EnableBusSupport=off
      mask Display:
      | port_label('input', 1, 'Active state');
      | port_label('input', 2, 'length');
      | port_label('input', 3, 'vel');
      | port_label('output', 1, 'tension');
      | disp('muscle model \n(S-Function)');
  T : Outport
  Spk : Outport  Port=2
  Fubglevant  twitch normal : Outport  Port=3
  wires:
  Constant6/1 -> muscle2/3
  motor neuron2/1 -> Scope19/1
  active state/1 -> Scope22/1, T/1, Fuglevand twitch/1
  motor neuron2/2 -> active state/1, Spk/1, Scope1/1
  synI/1 -> motor neuron2/1
  Lce/1 -> muscle2/2
  Fuglevand twitch/1 -> Fubglevant  twitch normal/1

== system motor_unit/Spastic/EMG reponse ==
  In1 : Inport
  Add1 : Sum
  Zero-Pole : ZeroPole  Zeros=[]  Poles=[-33 -33]  Gain=[2]
  Zero-Pole1 : ZeroPole  Zeros=[]  Poles=[-33 -33 -33]  Gain=[-2 * 33]
  Out1 : Outport
  wires:
  In1/1 -> Zero-Pole1/1, Zero-Pole/1
  Add1/1 -> Out1/1
  Zero-Pole1/1 -> Add1/2
  Zero-Pole/1 -> Add1/1

== system motor_unit/Spastic/EMG reponse1 ==
  In1 : Inport
  Add1 : Sum
  Zero-Pole : ZeroPole  Zeros=[]  Poles=[-33 -33]  Gain=[2]
  Zero-Pole1 : ZeroPole  Zeros=[]  Poles=[-33 -33 -33]  Gain=[-2 * 33]
  Out1 : Outport
  wires:
  In1/1 -> Zero-Pole1/1, Zero-Pole/1
  Add1/1 -> Out1/1
  Zero-Pole1/1 -> Add1/2
  Zero-Pole/1 -> Add1/1

== system motor_unit/Spastic/EMG response ==
  In1 : Inport
  Add2 : Sum
  Zero-Pole2 : ZeroPole  Zeros=[]  Poles=[-33 -33]  Gain=[2]
  Zero-Pole3 : ZeroPole  Zeros=[]  Poles=[-33 -33 -33]  Gain=[-2 * 33]
  Out1 : Outport
  wires:
  Add2/1 -> Out1/1
  In1/1 -> Zero-Pole3/1, Zero-Pole2/1
  Zero-Pole2/1 -> Add2/1
  Zero-Pole3/1 -> Add2/2

== system motor_unit/Spastic/Lowpass Filter ==
  In : Inport
  Generated Filter Block : dsparch4/Digital Filter  Tag=BlockMethodSubSystem  TypePopup=FIR (all zeros)  IIRFiltStruct=Direct form II transposed  AllPoleFiltStruct=Direct form  FIRFiltStruct=Direct form  CoeffSource=Specify via dialog  NumCoeffs=[0.000821343113298559 0.000860441837741389 0.00116507777294478 0.00139896051971534 0.00148073798259756 0.00133051719232521 0.000881379928818246 9.39666659446496e-05 -0.00102427649336678 -0.00241508381296073 -0.00396005761838719 -0.00548791113381279 -0.00678957165103652 -0.0076430176358472 -0.00784363593055865 -0.00724034355165257 -0.005767373855361 -0.00347179427273649 -0.000526738025008324 0.00277189505493066 0.00602772399348037 0.00878384411363102 0.0105793849551558 0.0110144101671425 0.00981730876000813 0.00690368741433792 0.00241805574190362 -0.00324979313849789 -0.00947842883556182 -0.0154612118882062 -0.0202815328070714 -0.0230109852998383 -0.0228194406688834 -0.0190843479651619 -0.0114852033107793 -7.04588646032898e-05 0.0147140504913441 0.032040450344853 0.0507590050669597 0.0694980891161205 0.0867940010093986 0.101236365407667 0.111612741087645 0.117035389882844 0.117035389882844 0.111612741087645 0.101236365407667 0.0867940010093986 0.0694980891161205 0.0507590050669597 0.032040450344853 0.0147140504913441 -7.04588646032898e-05 -0.0114852033107793 -0.0190843479651619 -0.0228194406688834 -0.0230109852998383 -0.0202815328070714 -0.0154612118882062 -0.00947842883556182 -0.00324979313849789 0.00241805574190362 0.00690368741433792 0.00981730876000813 0.0110144101671425 0.0105793849551558 0.00878384411363102 0.00602772399348037 0.00277189505493066 -0.000526738025008324 -0.00347179427273649 -0.005767373855361 -0.00724034355165257 -0.00784363593055865 -0.0076430176358472 -0.00678957165103652 -0.00548791113381279 -0.00396005761838719 -0.00241508381296073 -0.00102427649336678 9.39666659446496e-05 0.000881379928818246 0.00133051719232521 0.00148073798259756 0.00139896051971534 0.00116507777294478 0.000860441837741389 0.000821343113298559]  DenCoeffs=[1 0.1]  BiQuadCoeffs=[1 0.3 0.4 1 0.1 0.2]  LatticeCoeffs=[0.2 0.4]  denIgnore=on  FiltPerSampPopup=One filter per frame  IC=0  ICnum=0  ICden=0  roundingMode=Floor  overflowMode=off  ScaleValues=1  scaleValueFracLength=14  stageInFracLength=15  stageOutFracLength=15  FilterSource=Specify via dialog  dfiltObjectName=dfilt.dffir([1 2 1])  InputProcessing=Columns as channels (frame based)
  Out : Outport
  wires:
  Generated Filter Block/1 -> Out/1
  In/1 -> Generated Filter Block/1

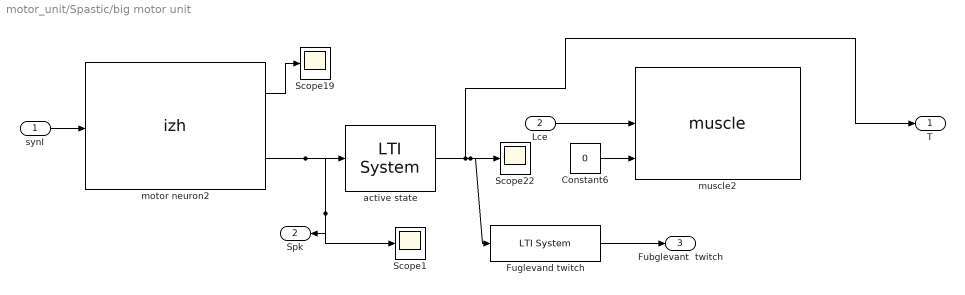
== system motor_unit/Spastic/big motor unit ==
  synI : Inport
  Lce : Inport  Port=2
  Constant6 : Constant  Value=0
  Fuglevand twitch : cstblocks/LTI System  sys=zpk([0], [0.93941 0.93941], 1*2.7183*0.001*0.93941/0.016, 0.001)  IC=[]
  Scope1 : Scope
      settings: TimeRange=0.4  YMin=-1000  YMax=5000  SaveName=ScopeData10
  Scope19 : Scope
      settings: SaveName=ScopeData19
  Scope22 : Scope
      settings: TimeRange=0.4  YMin=-1000  YMax=5000  SaveName=ScopeData22
  active state : cstblocks/LTI System  sys=0*zpk([0], A_rise, mag1, T) + zpk([0], exp(-T/0.04), mag2*8, T)  IC=[]
  motor neuron2 : S-Function  FunctionName=izh  Parameters=[0.02 0.2 -65.0 6.0 30.0 0.8] [-70.0 -14.0]  EnableBusSupport=off
      mask Display:
      | port_label('input', 1, 'syn curr');
      | port_label('output', 1, 'action potential');
      | port_label('output', 2, 'spike');
      | disp('Izhi Neuron \n(S-Function)')
  muscle2 : S-Function  FunctionName=muscle  Parameters=[136.0 75.0 50.0] [0]  EnableBusSupport=off
      mask Display:
      | port_label('input', 1, 'Active state');
      | port_label('input', 2, 'length');
      | port_label('input', 3, 'vel');
      | port_label('output', 1, 'tension');
      | disp('muscle model \n(S-Function)');
  T : Outport
  Spk : Outport  Port=2
  Fubglevant  twitch : Outport  Port=3
  wires:
  Lce/1 -> muscle2/2
  synI/1 -> motor neuron2/1
  motor neuron2/2 -> Scope1/1, Spk/1, active state/1
  active state/1 -> T/1, Scope22/1, Fuglevand twitch/1
  motor neuron2/1 -> Scope19/1
  Constant6/1 -> muscle2/3
  Fuglevand twitch/1 -> Fubglevant  twitch/1

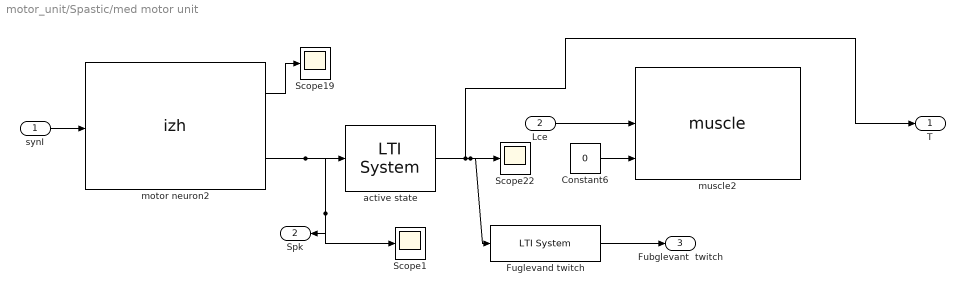
== system motor_unit/Spastic/med motor unit ==
  synI : Inport
  Lce : Inport  Port=2
  Constant6 : Constant  Value=0
  Fuglevand twitch : cstblocks/LTI System  sys=zpk([0], [0.93941 0.93941], 1*2.7183*0.001*0.93941/0.016, 0.001)  IC=[]
  Scope1 : Scope
      settings: TimeRange=0.4  YMin=-1000  YMax=5000  SaveName=ScopeData10
  Scope19 : Scope
      settings: SaveName=ScopeData19
  Scope22 : Scope
      settings: TimeRange=0.4  YMin=-1000  YMax=5000  SaveName=ScopeData22
  active state : cstblocks/LTI System  sys="0*zpk([0], A_rise, mag1, T) + zpk([0], exp(-T/0.06),  mag2*3.5, T)"  IC=[]
  motor neuron2 : S-Function  FunctionName=izh  Parameters=[0.02 0.2 -65.0 6.0 30.0 0.9] [-70.0 -14.0]  EnableBusSupport=off
      mask Display:
      | port_label('input', 1, 'syn curr');
      | port_label('output', 1, 'action potential');
      | port_label('output', 2, 'spike');
      | disp('Izhi Neuron \n(S-Function)')
  muscle2 : S-Function  FunctionName=muscle  Parameters=[136.0 75.0 50.0] [0]  EnableBusSupport=off
      mask Display:
      | port_label('input', 1, 'Active state');
      | port_label('input', 2, 'length');
      | port_label('input', 3, 'vel');
      | port_label('output', 1, 'tension');
      | disp('muscle model \n(S-Function)');
  T : Outport
  Spk : Outport  Port=2
  Fubglevant  twitch : Outport  Port=3
  wires:
  Fuglevand twitch/1 -> Fubglevant  twitch/1
  Constant6/1 -> muscle2/3
  motor neuron2/1 -> Scope19/1
  active state/1 -> Fuglevand twitch/1, Scope22/1, T/1
  motor neuron2/2 -> active state/1, Spk/1, Scope1/1
  synI/1 -> motor neuron2/1
  Lce/1 -> muscle2/2

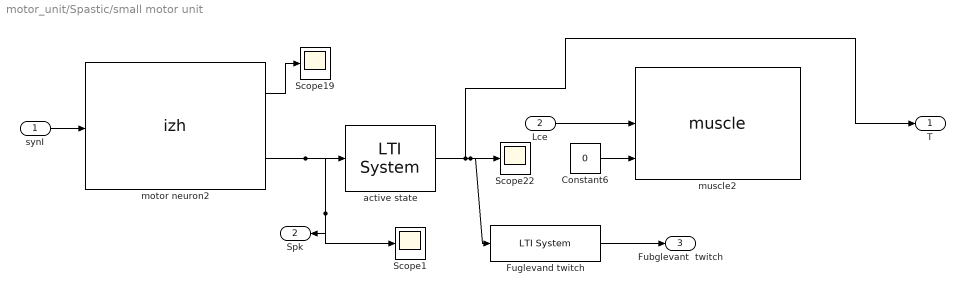
== system motor_unit/Spastic/small motor unit ==
  synI : Inport
  Lce : Inport  Port=2
  Constant6 : Constant  Value=0
  Fuglevand twitch : cstblocks/LTI System  sys=zpk([0], [0.93941 0.93941], 1*2.7183*0.001*0.93941/0.016, 0.001)  IC=[]
  Scope1 : Scope
      settings: TimeRange=0.4  YMin=-1000  YMax=5000  SaveName=ScopeData10
  Scope19 : Scope
      settings: SaveName=ScopeData19
  Scope22 : Scope
      settings: TimeRange=0.4  YMin=-1000  YMax=5000  SaveName=ScopeData22
  active state : cstblocks/LTI System  sys="0*zpk([0], A_rise, mag1, T) + zpk([0], exp(-T/0.09),  mag2*1, T)"  IC=[]
  motor neuron2 : S-Function  FunctionName=izh  Parameters=[0.02 0.2 -65.0 6.0 30.0 1.0] [-70.0 -14.0]  EnableBusSupport=off
      mask Display:
      | port_label('input', 1, 'syn curr');
      | port_label('output', 1, 'action potential');
      | port_label('output', 2, 'spike');
      | disp('Izhi Neuron \n(S-Function)')
  muscle2 : S-Function  FunctionName=muscle  Parameters=[136.0 75.0 50.0] [0]  EnableBusSupport=off
      mask Display:
      | port_label('input', 1, 'Active state');
      | port_label('input', 2, 'length');
      | port_label('input', 3, 'vel');
      | port_label('output', 1, 'tension');
      | disp('muscle model \n(S-Function)');
  T : Outport
  Spk : Outport  Port=2
  Fubglevant  twitch : Outport  Port=3
  wires:
  Lce/1 -> muscle2/2
  synI/1 -> motor neuron2/1
  motor neuron2/2 -> Scope1/1, Spk/1, active state/1
  active state/1 -> T/1, Scope22/1, Fuglevand twitch/1
  motor neuron2/1 -> Scope19/1
  Constant6/1 -> muscle2/3
  Fuglevand twitch/1 -> Fubglevant  twitch/1

== system motor_unit/Spastic1/EMG reponse ==
  In1 : Inport
  Add1 : Sum
  Zero-Pole : ZeroPole  Zeros=[]  Poles=[-33 -33]  Gain=[2]
  Zero-Pole1 : ZeroPole  Zeros=[]  Poles=[-33 -33 -33]  Gain=[-2 * 33]
  Out1 : Outport
  wires:
  Zero-Pole/1 -> Add1/1
  Zero-Pole1/1 -> Add1/2
  Add1/1 -> Out1/1
  In1/1 -> Zero-Pole/1, Zero-Pole1/1

== system motor_unit/Spastic1/EMG reponse1 ==
  In1 : Inport
  Add1 : Sum
  Zero-Pole : ZeroPole  Zeros=[]  Poles=[-33 -33]  Gain=[2]
  Zero-Pole1 : ZeroPole  Zeros=[]  Poles=[-33 -33 -33]  Gain=[-2 * 33]
  Out1 : Outport
  wires:
  Zero-Pole/1 -> Add1/1
  Zero-Pole1/1 -> Add1/2
  Add1/1 -> Out1/1
  In1/1 -> Zero-Pole/1, Zero-Pole1/1

== system motor_unit/Spastic1/EMG response ==
  In1 : Inport
  Add2 : Sum
  Zero-Pole2 : ZeroPole  Zeros=[]  Poles=[-33 -33]  Gain=[2]
  Zero-Pole3 : ZeroPole  Zeros=[]  Poles=[-33 -33 -33]  Gain=[-2 * 33]
  Out1 : Outport
  wires:
  Zero-Pole3/1 -> Add2/2
  Zero-Pole2/1 -> Add2/1
  In1/1 -> Zero-Pole2/1, Zero-Pole3/1
  Add2/1 -> Out1/1

== system motor_unit/Spastic1/Lowpass Filter ==
  In : Inport
  Generated Filter Block : dsparch4/Digital Filter  Tag=BlockMethodSubSystem  TypePopup=FIR (all zeros)  IIRFiltStruct=Direct form II transposed  AllPoleFiltStruct=Direct form  FIRFiltStruct=Direct form  CoeffSource=Specify via dialog  NumCoeffs=[0.000821343113298559 0.000860441837741389 0.00116507777294478 0.00139896051971534 0.00148073798259756 0.00133051719232521 0.000881379928818246 9.39666659446496e-05 -0.00102427649336678 -0.00241508381296073 -0.00396005761838719 -0.00548791113381279 -0.00678957165103652 -0.0076430176358472 -0.00784363593055865 -0.00724034355165257 -0.005767373855361 -0.00347179427273649 -0.000526738025008324 0.00277189505493066 0.00602772399348037 0.00878384411363102 0.0105793849551558 0.0110144101671425 0.00981730876000813 0.00690368741433792 0.00241805574190362 -0.00324979313849789 -0.00947842883556182 -0.0154612118882062 -0.0202815328070714 -0.0230109852998383 -0.0228194406688834 -0.0190843479651619 -0.0114852033107793 -7.04588646032898e-05 0.0147140504913441 0.032040450344853 0.0507590050669597 0.0694980891161205 0.0867940010093986 0.101236365407667 0.111612741087645 0.117035389882844 0.117035389882844 0.111612741087645 0.101236365407667 0.0867940010093986 0.0694980891161205 0.0507590050669597 0.032040450344853 0.0147140504913441 -7.04588646032898e-05 -0.0114852033107793 -0.0190843479651619 -0.0228194406688834 -0.0230109852998383 -0.0202815328070714 -0.0154612118882062 -0.00947842883556182 -0.00324979313849789 0.00241805574190362 0.00690368741433792 0.00981730876000813 0.0110144101671425 0.0105793849551558 0.00878384411363102 0.00602772399348037 0.00277189505493066 -0.000526738025008324 -0.00347179427273649 -0.005767373855361 -0.00724034355165257 -0.00784363593055865 -0.0076430176358472 -0.00678957165103652 -0.00548791113381279 -0.00396005761838719 -0.00241508381296073 -0.00102427649336678 9.39666659446496e-05 0.000881379928818246 0.00133051719232521 0.00148073798259756 0.00139896051971534 0.00116507777294478 0.000860441837741389 0.000821343113298559]  DenCoeffs=[1 0.1]  BiQuadCoeffs=[1 0.3 0.4 1 0.1 0.2]  LatticeCoeffs=[0.2 0.4]  denIgnore=on  FiltPerSampPopup=One filter per frame  IC=0  ICnum=0  ICden=0  roundingMode=Floor  overflowMode=off  ScaleValues=1  scaleValueFracLength=14  stageInFracLength=15  stageOutFracLength=15  FilterSource=Specify via dialog  dfiltObjectName=dfilt.dffir([1 2 1])  InputProcessing=Columns as channels (frame based)
  Out : Outport
  wires:
  In/1 -> Generated Filter Block/1
  Generated Filter Block/1 -> Out/1

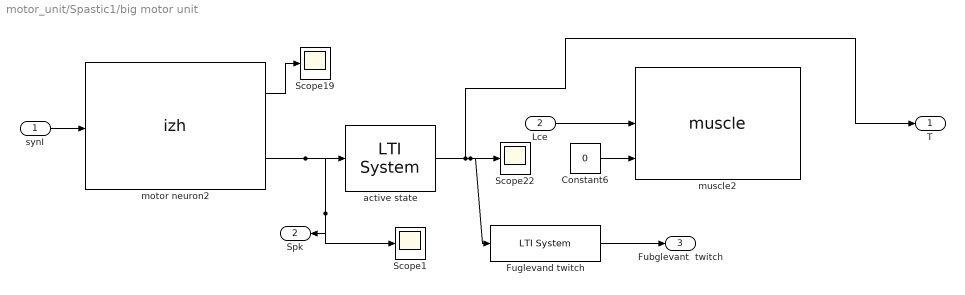
== system motor_unit/Spastic1/big motor unit ==
  synI : Inport
  Lce : Inport  Port=2
  Constant6 : Constant  Value=0
  Fuglevand twitch : cstblocks/LTI System  sys=zpk([0], [0.93941 0.93941], 1*2.7183*0.001*0.93941/0.016, 0.001)  IC=[]
  Scope1 : Scope
      settings: TimeRange=0.4  YMin=-1000  YMax=5000  SaveName=ScopeData10
  Scope19 : Scope
      settings: SaveName=ScopeData19
  Scope22 : Scope
      settings: TimeRange=0.4  YMin=-1000  YMax=5000  SaveName=ScopeData22
  active state : cstblocks/LTI System  sys=0*zpk([0], A_rise, mag1, T) + zpk([0], exp(-T/0.04), mag2*8, T)  IC=[]
  motor neuron2 : S-Function  FunctionName=izh  Parameters=[0.02 0.2 -65.0 6.0 30.0 0.8] [-70.0 -14.0]  EnableBusSupport=off
      mask Display:
      | port_label('input', 1, 'syn curr');
      | port_label('output', 1, 'action potential');
      | port_label('output', 2, 'spike');
      | disp('Izhi Neuron \n(S-Function)')
  muscle2 : S-Function  FunctionName=muscle  Parameters=[136.0 75.0 50.0] [0]  EnableBusSupport=off
      mask Display:
      | port_label('input', 1, 'Active state');
      | port_label('input', 2, 'length');
      | port_label('input', 3, 'vel');
      | port_label('output', 1, 'tension');
      | disp('muscle model \n(S-Function)');
  T : Outport
  Spk : Outport  Port=2
  Fubglevant  twitch : Outport  Port=3
  wires:
  Fuglevand twitch/1 -> Fubglevant  twitch/1
  Constant6/1 -> muscle2/3
  motor neuron2/1 -> Scope19/1
  active state/1 -> Fuglevand twitch/1, Scope22/1, T/1
  motor neuron2/2 -> active state/1, Spk/1, Scope1/1
  synI/1 -> motor neuron2/1
  Lce/1 -> muscle2/2

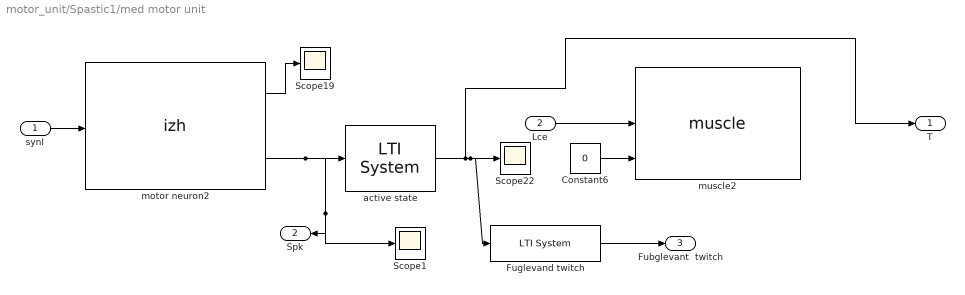
== system motor_unit/Spastic1/med motor unit ==
  synI : Inport
  Lce : Inport  Port=2
  Constant6 : Constant  Value=0
  Fuglevand twitch : cstblocks/LTI System  sys=zpk([0], [0.93941 0.93941], 1*2.7183*0.001*0.93941/0.016, 0.001)  IC=[]
  Scope1 : Scope
      settings: TimeRange=0.4  YMin=-1000  YMax=5000  SaveName=ScopeData10
  Scope19 : Scope
      settings: SaveName=ScopeData19
  Scope22 : Scope
      settings: TimeRange=0.4  YMin=-1000  YMax=5000  SaveName=ScopeData22
  active state : cstblocks/LTI System  sys="0*zpk([0], A_rise, mag1, T) + zpk([0], exp(-T/0.06),  mag2*3.5, T)"  IC=[]
  motor neuron2 : S-Function  FunctionName=izh  Parameters=[0.02 0.2 -65.0 6.0 30.0 0.9] [-70.0 -14.0]  EnableBusSupport=off
      mask Display:
      | port_label('input', 1, 'syn curr');
      | port_label('output', 1, 'action potential');
      | port_label('output', 2, 'spike');
      | disp('Izhi Neuron \n(S-Function)')
  muscle2 : S-Function  FunctionName=muscle  Parameters=[136.0 75.0 50.0] [0]  EnableBusSupport=off
      mask Display:
      | port_label('input', 1, 'Active state');
      | port_label('input', 2, 'length');
      | port_label('input', 3, 'vel');
      | port_label('output', 1, 'tension');
      | disp('muscle model \n(S-Function)');
  T : Outport
  Spk : Outport  Port=2
  Fubglevant  twitch : Outport  Port=3
  wires:
  Lce/1 -> muscle2/2
  synI/1 -> motor neuron2/1
  motor neuron2/2 -> Scope1/1, Spk/1, active state/1
  active state/1 -> T/1, Scope22/1, Fuglevand twitch/1
  motor neuron2/1 -> Scope19/1
  Constant6/1 -> muscle2/3
  Fuglevand twitch/1 -> Fubglevant  twitch/1

== system motor_unit/Spastic1/small motor unit ==
  synI : Inport
  Lce : Inport  Port=2
  Constant6 : Constant  Value=0
  Fuglevand twitch : cstblocks/LTI System  sys=zpk([0], [0.93941 0.93941], 1*2.7183*0.001*0.93941/0.016, 0.001)  IC=[]
  Scope1 : Scope
      settings: TimeRange=0.4  YMin=-1000  YMax=5000  SaveName=ScopeData10
  Scope19 : Scope
      settings: SaveName=ScopeData19
  Scope22 : Scope
      settings: TimeRange=0.4  YMin=-1000  YMax=5000  SaveName=ScopeData22
  active state : cstblocks/LTI System  sys="0*zpk([0], A_rise, mag1, T) + zpk([0], exp(-T/0.09),  mag2*1, T)"  IC=[]
  motor neuron2 : S-Function  FunctionName=izh  Parameters=[0.02 0.2 -65.0 6.0 30.0 1.0] [-70.0 -14.0]  EnableBusSupport=off
      mask Display:
      | port_label('input', 1, 'syn curr');
      | port_label('output', 1, 'action potential');
      | port_label('output', 2, 'spike');
      | disp('Izhi Neuron \n(S-Function)')
  muscle2 : S-Function  FunctionName=muscle  Parameters=[136.0 75.0 50.0] [0]  EnableBusSupport=off
      mask Display:
      | port_label('input', 1, 'Active state');
      | port_label('input', 2, 'length');
      | port_label('input', 3, 'vel');
      | port_label('output', 1, 'tension');
      | disp('muscle model \n(S-Function)');
  T : Outport
  Spk : Outport  Port=2
  Fubglevant  twitch : Outport  Port=3
  wires:
  Fuglevand twitch/1 -> Fubglevant  twitch/1
  Constant6/1 -> muscle2/3
  motor neuron2/1 -> Scope19/1
  active state/1 -> Fuglevand twitch/1, Scope22/1, T/1
  motor neuron2/2 -> active state/1, Spk/1, Scope1/1
  synI/1 -> motor neuron2/1
  Lce/1 -> muscle2/2
